simulink model "CruiseControl"  (R2020a)
settings: Solver=VariableStepAuto  StartTime=0.0  StopTime=120.0  RelTol=1e-3
PostLoadFcn:
  | m=1000;
  | b=50;
  | u=500;
model workspace (MAT data in the model file):
  Kd = 10
  Ki = 40
  Kp = 800
settings Model: DataDictionary=DataDictionary.sldd  Creator=Hp  LastModifiedBy=Hp

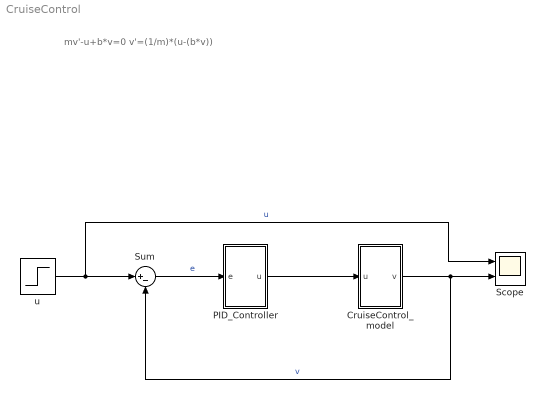
== system CruiseControl ==
  note: mv'-u+b*v=0
      | v'=(1/m)*(u-(b*v))
  CruiseControl_model : Subsystem
  PID_Controller : Subsystem
  Scope : Scope  NumInputPorts=2
  Sum : Sum  Inputs=|+-
  u : Step  Time=0  After=u  SampleTime=0
  wires:
  CruiseControl_model/1(v) -> Sum/2, Scope/2  "v"
  u/1 -> Scope/1, Sum/1  "u"
  Sum/1 -> PID_Controller/1(e)  "e"
  PID_Controller/1(u) -> CruiseControl_model/1(u)

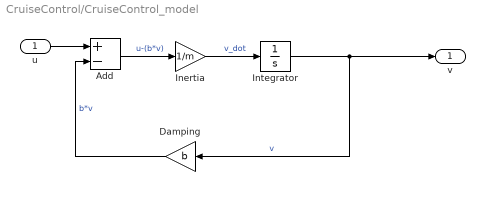
== system CruiseControl/CruiseControl_model ==
  u : Inport
  Add : Sum  Inputs=+-
  Damping : Gain  Gain=b
  Inertia : Gain  Gain=1/m
  Integrator : Integrator
  v : Outport
  wires:
  Damping/1 -> Add/2  "b*v"
  Inertia/1 -> Integrator/1  "v_dot"
  Integrator/1 -> v/1, Damping/1  "v"
  Add/1 -> Inertia/1  "u-(b*v)"
  u/1 -> Add/1

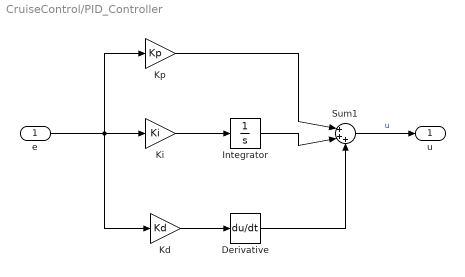
== system CruiseControl/PID_Controller ==
  e : Inport
  Derivative : Derivative
  Integrator : Integrator
  Kd : Gain  Gain=Kd
  Ki : Gain  Gain=Ki
  Kp : Gain  Gain=Kp
  Sum1 : Sum  Inputs=|+++
  u : Outport
  wires:
  Integrator/1 -> Sum1/2
  Kp/1 -> Sum1/1
  Ki/1 -> Integrator/1
  e/1 -> Kd/1, Kp/1, Ki/1
  Kd/1 -> Derivative/1
  Derivative/1 -> Sum1/3
  Sum1/1 -> u/1  "u"
